simulink model "Controllo_Totale"  (R2013a)
settings: Solver=ode45  StartTime=0.0  StopTime=inf  RelTol=1e-3
undefined symbols (not defined in the file or in its folder): d, r
libraries: simulink x9, dspsigops x8, arduino_io_lib x6, xpcseriallib x2, dspnetwork x2
settings Model: Creator=Francesco  LastModifiedBy=Francesco

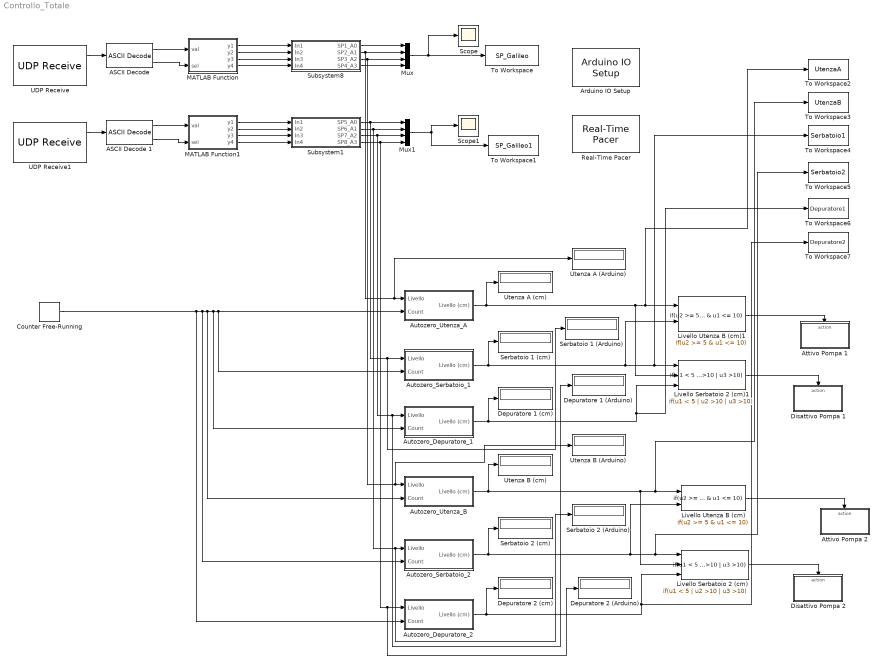
== system Controllo_Totale ==
  "ASCII Decode " : xpcseriallib/ASCII Decode   format=%d*%d\r  nvars=2  vartypes={ }
  ASCII Decode 1 : xpcseriallib/ASCII Decode   format=%d*%d\r  nvars=2  vartypes={ }
  Arduino IO Setup : arduino_io_lib/Arduino IO Setup  Priority=3  arduinoVar=Temporary arduino variable: Arduino1  workspaceVarName=a  comPort=COM3
  Attivo Pompa 1 : Subsystem  TreatAsAtomicUnit=on
  Attivo Pompa 2 : Subsystem  TreatAsAtomicUnit=on
  Autozero_Depuratore_1 : Subsystem
  Autozero_Depuratore_2 : Subsystem
  Autozero_Serbatoio_1 : Subsystem
  Autozero_Serbatoio_2 : Subsystem
  Autozero_Utenza_A : Subsystem
  Autozero_Utenza_B : Subsystem
  Counter Free-Running : simulink/Sources/Counter Free-Running  NumBits=32  tsamp=-1
  Depuratore 1 (Arduino) : Display
  Depuratore 1 (cm) : Display
  Depuratore 2 (Arduino) : Display
  Depuratore 2 (cm) : Display
  Disattivo Pompa 1 : Subsystem  TreatAsAtomicUnit=on
  Disattivo Pompa 2 : Subsystem  TreatAsAtomicUnit=on
  Livello Serbatoio 2 (cm) : If  NumInputs=3  IfExpression=u1 < 5 | u2 >10 | u3 >10  ShowElse=off
  Livello Serbatoio 2 (cm)1 : If  NumInputs=3  IfExpression=u1 < 5 | u2 >10 | u3 >10  ShowElse=off
  Livello Utenza B (cm) : If  NumInputs=2  IfExpression=u2 >= 5 & u1 <= 10  ShowElse=off
  Livello Utenza B (cm)1 : If  NumInputs=2  IfExpression=u2 >= 5 & u1 <= 10  ShowElse=off
  MATLAB Function : MATLAB Function  TreatAsAtomicUnit=on
  MATLAB Function1 : MATLAB Function  TreatAsAtomicUnit=on
  Mux : Mux
  Mux1 : Mux
  Real-Time Pacer : arduino_io_lib/Real-Time Pacer  simTimePerRealTime=1
  Scope : Scope
      settings: TimeRange=50  YMin=0  YMax=475
  Scope1 : Scope
      settings: TimeRange=50  YMin=327.5  YMax=360
  Serbatoio 1 (Arduino) : Display
  Serbatoio 1 (cm) : Display
  Serbatoio 2 (Arduino) : Display
  Serbatoio 2 (cm) : Display
  Subsystem1 : Subsystem
  Subsystem8 : Subsystem
  To Workspace : ToWorkspace  VariableName=SP_Galileo  SampleTime=-1  SaveFormat=Timeseries
  To Workspace1 : ToWorkspace  VariableName=SP_Galileo1  SampleTime=-1  SaveFormat=Timeseries
  To Workspace2 : ToWorkspace  VariableName=UtenzaA  SampleTime=-1
  To Workspace3 : ToWorkspace  VariableName=UtenzaB  SampleTime=-1
  To Workspace4 : ToWorkspace  VariableName=Serbatoio1  SampleTime=-1
  To Workspace5 : ToWorkspace  VariableName=Serbatoio2  SampleTime=-1
  To Workspace6 : ToWorkspace  VariableName=Depuratore1  SampleTime=-1
  To Workspace7 : ToWorkspace  VariableName=Depuratore2  SampleTime=-1
  UDP Receive : dspnetwork/UDP Receive  localURL='0.0.0.0'  localPort=4040  remoteURL='192.168.2.4'  remotePort=-1  recvBufferSize=1  dims=5  signalDatatype=uint8  isVarSize=off  showBlockingTime=on  blockingTime=inf  sampletime=1  blockPlatform=LINUX
  UDP Receive1 : dspnetwork/UDP Receive  localURL='0.0.0.0'  localPort=4040  remoteURL='192.168.2.6'  remotePort=-1  recvBufferSize=1  dims=5  signalDatatype=uint8  isVarSize=off  showBlockingTime=on  blockingTime=inf  sampletime=1  blockPlatform=LINUX
  Utenza A (Arduino) : Display
  Utenza A (cm) : Display
  Utenza B (Arduino) : Display
  Utenza B (cm) : Display
  wires:
  UDP Receive/1 -> "ASCII Decode "/1
  "ASCII Decode "/1 -> MATLAB Function/1(val)
  "ASCII Decode "/2 -> MATLAB Function/2(sel)
  Mux/1 -> To Workspace/1, Scope/1
  UDP Receive1/1 -> ASCII Decode 1/1
  ASCII Decode 1/1 -> MATLAB Function1/1(val)
  ASCII Decode 1/2 -> MATLAB Function1/2(sel)
  Mux1/1 -> To Workspace1/1, Scope1/1
  MATLAB Function/1(y1) -> Subsystem8/1(In1)
  MATLAB Function/2(y2) -> Subsystem8/2(In2)
  MATLAB Function/3(y3) -> Subsystem8/3(In3)
  MATLAB Function/4(y4) -> Subsystem8/4(In4)
  Subsystem8/1(SP1_A0) -> Mux/1
  Subsystem8/2(SP2_A1) -> Utenza A (Arduino)/1, Autozero_Utenza_A/1(Livello), Mux/2
  Subsystem8/3(SP3_A2) -> Utenza B (Arduino)/1, Autozero_Utenza_B/1(Livello), Mux/3
  Subsystem8/4(SP4_A3) -> Mux/4
  MATLAB Function1/1(y1) -> Subsystem1/1(In1)
  MATLAB Function1/2(y2) -> Subsystem1/2(In2)
  MATLAB Function1/3(y3) -> Subsystem1/3(In3)
  MATLAB Function1/4(y4) -> Subsystem1/4(In4)
  Subsystem1/1(SP5_A0) -> Autozero_Serbatoio_1/1(Livello), Serbatoio 1 (Arduino)/1, Mux1/1
  Subsystem1/2(SP6_A1) -> Serbatoio 2 (Arduino)/1, Autozero_Serbatoio_2/1(Livello), Mux1/2
  Subsystem1/3(SP7_A2) -> Depuratore 1 (Arduino)/1, Autozero_Depuratore_1/1(Livello), Mux1/3
  Subsystem1/4(SP8_A3) -> Depuratore 2 (Arduino)/1, Autozero_Depuratore_2/1(Livello), Mux1/4
  Autozero_Utenza_B/1(Livello (cm)) -> Livello Serbatoio 2 (cm)/2, To Workspace3/1, Livello Utenza B (cm)/1, Utenza B (cm)/1
  Counter Free-Running/1 -> Autozero_Depuratore_2/2(Count), Autozero_Utenza_A/2(Count), Autozero_Serbatoio_1/2(Count), Autozero_Depuratore_1/2(Count), Autozero_Utenza_B/2(Count), Autozero_Serbatoio_2/2(Count)
  Autozero_Serbatoio_2/1(Livello (cm)) -> Livello Utenza B (cm)/2, To Workspace5/1, Livello Serbatoio 2 (cm)/1, Serbatoio 2 (cm)/1
  Autozero_Depuratore_2/1(Livello (cm)) -> To Workspace7/1, Livello Serbatoio 2 (cm)/3, Depuratore 2 (cm)/1
  Livello Utenza B (cm)/1 -> Attivo Pompa 2/Action
  Livello Serbatoio 2 (cm)/1 -> Disattivo Pompa 2/Action
  Livello Utenza B (cm)1/1 -> Attivo Pompa 1/Action
  Livello Serbatoio 2 (cm)1/1 -> Disattivo Pompa 1/Action
  Autozero_Utenza_A/1(Livello (cm)) -> Utenza A (cm)/1, Livello Serbatoio 2 (cm)1/2, To Workspace2/1, Livello Utenza B (cm)1/1
  Autozero_Serbatoio_1/1(Livello (cm)) -> Serbatoio 1 (cm)/1, Livello Utenza B (cm)1/2, To Workspace4/1, Livello Serbatoio 2 (cm)1/1
  Autozero_Depuratore_1/1(Livello (cm)) -> Depuratore 1 (cm)/1, To Workspace6/1, Livello Serbatoio 2 (cm)1/3

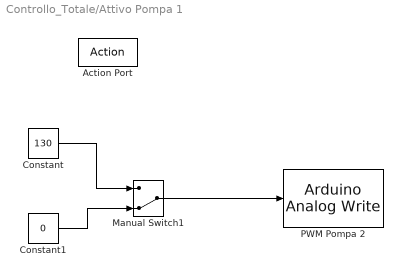
== system Controllo_Totale/Attivo Pompa 1 ==
  Action Port : ActionPort  ActionType=then
  Constant : Constant  Value=130
  Constant1 : Constant  Value=0  SampleTime=1
  Manual Switch1 : ManualSwitch  CurrentSetting=0
  PWM Pompa 2 : arduino_io_lib/Arduino Analog Write  arduinoVar=Temporary arduino variable: Arduino1  arduinoPin=5  T=1
  wires:
  Constant/1 -> Manual Switch1/1
  Constant1/1 -> Manual Switch1/2
  Manual Switch1/1 -> PWM Pompa 2/1

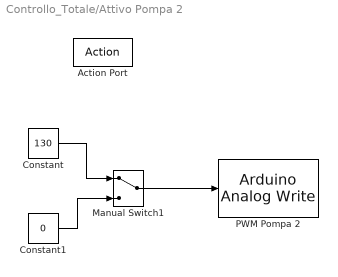
== system Controllo_Totale/Attivo Pompa 2 ==
  Action Port : ActionPort  ActionType=then
  Constant : Constant  Value=130
  Constant1 : Constant  Value=0  SampleTime=1
  Manual Switch1 : ManualSwitch
  PWM Pompa 2 : arduino_io_lib/Arduino Analog Write  arduinoVar=Temporary arduino variable: Arduino1  arduinoPin=6  T=1
  wires:
  Constant/1 -> Manual Switch1/1
  Constant1/1 -> Manual Switch1/2
  Manual Switch1/1 -> PWM Pompa 2/1

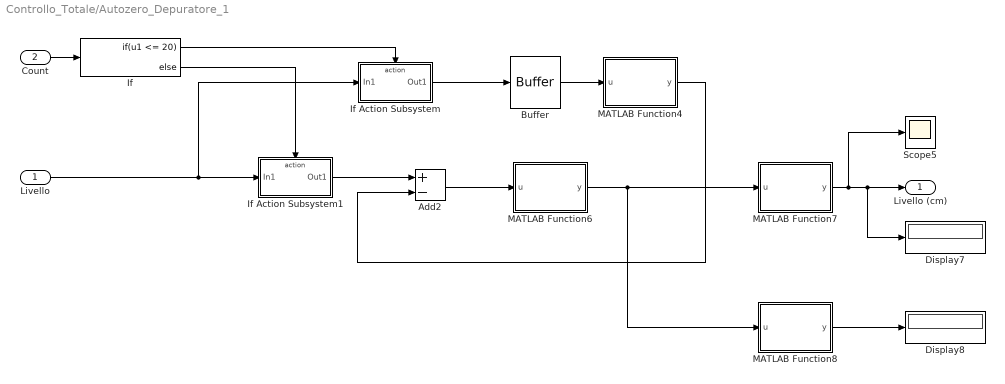
== system Controllo_Totale/Autozero_Depuratore_1 ==
  Livello : Inport
  Count : Inport  Port=2
  Add2 : Sum  Inputs=+-
  Buffer : Buffer  N=20  TreatMby1Signals=One channel
  Display7 : Display
  Display8 : Display
  If : If  IfExpression=u1 <= 20
  If Action Subsystem : Subsystem  TreatAsAtomicUnit=on
  If Action Subsystem1 : Subsystem  TreatAsAtomicUnit=on
  MATLAB Function4 : MATLAB Function  TreatAsAtomicUnit=on
  MATLAB Function6 : MATLAB Function  TreatAsAtomicUnit=on
  MATLAB Function7 : MATLAB Function  TreatAsAtomicUnit=on
  MATLAB Function8 : MATLAB Function  TreatAsAtomicUnit=on
  Scope5 : Scope
      settings: SaveName=ScopeData4
  Livello (cm) : Outport
  wires:
  Buffer/1 -> MATLAB Function4/1(u)
  MATLAB Function4/1(y) -> Add2/2
  If/1 -> If Action Subsystem/Action
  If/2 -> If Action Subsystem1/Action
  Add2/1 -> MATLAB Function6/1(u)
  MATLAB Function6/1(y) -> MATLAB Function8/1(u), MATLAB Function7/1(u)
  MATLAB Function8/1(y) -> Display8/1
  If Action Subsystem/1(Out1) -> Buffer/1
  MATLAB Function7/1(y) -> Display7/1, Livello (cm)/1, Scope5/1
  Count/1 -> If/1
  If Action Subsystem1/1(Out1) -> Add2/1
  Livello/1 -> If Action Subsystem/1(In1), If Action Subsystem1/1(In1)

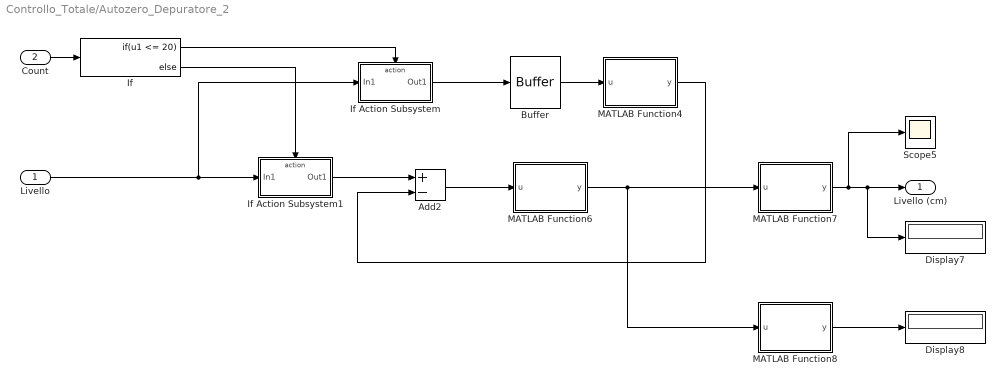
== system Controllo_Totale/Autozero_Depuratore_2 ==
  Livello : Inport
  Count : Inport  Port=2
  Add2 : Sum  Inputs=+-
  Buffer : Buffer  N=20  TreatMby1Signals=One channel
  Display7 : Display
  Display8 : Display
  If : If  IfExpression=u1 <= 20
  If Action Subsystem : Subsystem  TreatAsAtomicUnit=on
  If Action Subsystem1 : Subsystem  TreatAsAtomicUnit=on
  MATLAB Function4 : MATLAB Function  TreatAsAtomicUnit=on
  MATLAB Function6 : MATLAB Function  TreatAsAtomicUnit=on
  MATLAB Function7 : MATLAB Function  TreatAsAtomicUnit=on
  MATLAB Function8 : MATLAB Function  TreatAsAtomicUnit=on
  Scope5 : Scope
      settings: SaveName=ScopeData7
  Livello (cm) : Outport
  wires:
  Buffer/1 -> MATLAB Function4/1(u)
  MATLAB Function4/1(y) -> Add2/2
  If/1 -> If Action Subsystem/Action
  If/2 -> If Action Subsystem1/Action
  Add2/1 -> MATLAB Function6/1(u)
  MATLAB Function6/1(y) -> MATLAB Function8/1(u), MATLAB Function7/1(u)
  MATLAB Function8/1(y) -> Display8/1
  If Action Subsystem/1(Out1) -> Buffer/1
  MATLAB Function7/1(y) -> Display7/1, Livello (cm)/1, Scope5/1
  Count/1 -> If/1
  If Action Subsystem1/1(Out1) -> Add2/1
  Livello/1 -> If Action Subsystem/1(In1), If Action Subsystem1/1(In1)

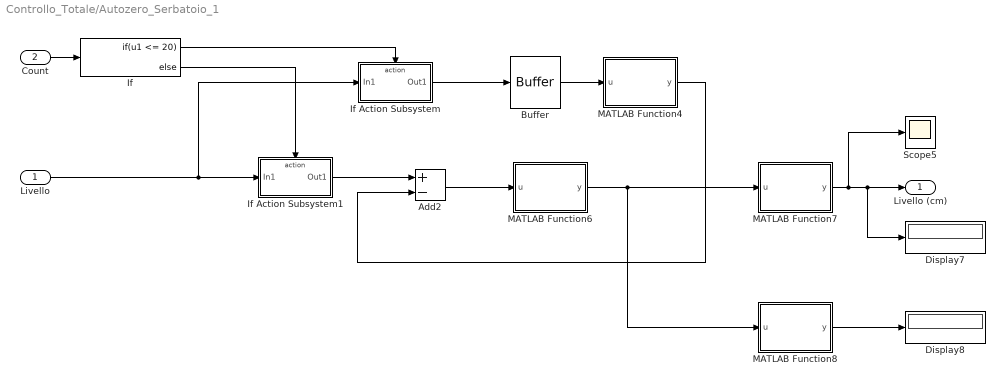
== system Controllo_Totale/Autozero_Serbatoio_1 ==
  Livello : Inport
  Count : Inport  Port=2
  Add2 : Sum  Inputs=+-
  Buffer : Buffer  N=20  TreatMby1Signals=One channel
  Display7 : Display
  Display8 : Display
  If : If  IfExpression=u1 <= 20
  If Action Subsystem : Subsystem  TreatAsAtomicUnit=on
  If Action Subsystem1 : Subsystem  TreatAsAtomicUnit=on
  MATLAB Function4 : MATLAB Function  TreatAsAtomicUnit=on
  MATLAB Function6 : MATLAB Function  TreatAsAtomicUnit=on
  MATLAB Function7 : MATLAB Function  TreatAsAtomicUnit=on
  MATLAB Function8 : MATLAB Function  TreatAsAtomicUnit=on
  Scope5 : Scope
      settings: SaveName=ScopeData2
  Livello (cm) : Outport
  wires:
  Buffer/1 -> MATLAB Function4/1(u)
  MATLAB Function4/1(y) -> Add2/2
  If/1 -> If Action Subsystem/Action
  If/2 -> If Action Subsystem1/Action
  Add2/1 -> MATLAB Function6/1(u)
  MATLAB Function6/1(y) -> MATLAB Function8/1(u), MATLAB Function7/1(u)
  MATLAB Function8/1(y) -> Display8/1
  If Action Subsystem/1(Out1) -> Buffer/1
  MATLAB Function7/1(y) -> Display7/1, Livello (cm)/1, Scope5/1
  Count/1 -> If/1
  If Action Subsystem1/1(Out1) -> Add2/1
  Livello/1 -> If Action Subsystem/1(In1), If Action Subsystem1/1(In1)

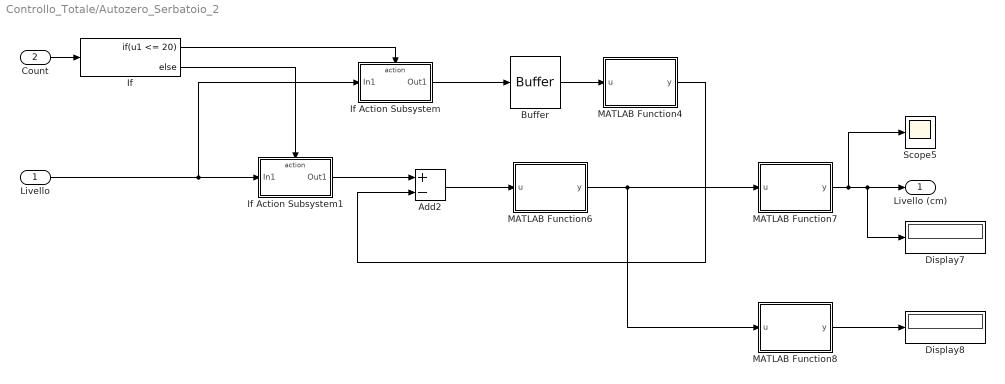
== system Controllo_Totale/Autozero_Serbatoio_2 ==
  Livello : Inport
  Count : Inport  Port=2
  Add2 : Sum  Inputs=+-
  Buffer : Buffer  N=20  TreatMby1Signals=One channel
  Display7 : Display
  Display8 : Display
  If : If  IfExpression=u1 <= 20
  If Action Subsystem : Subsystem  TreatAsAtomicUnit=on
  If Action Subsystem1 : Subsystem  TreatAsAtomicUnit=on
  MATLAB Function4 : MATLAB Function  TreatAsAtomicUnit=on
  MATLAB Function6 : MATLAB Function  TreatAsAtomicUnit=on
  MATLAB Function7 : MATLAB Function  TreatAsAtomicUnit=on
  MATLAB Function8 : MATLAB Function  TreatAsAtomicUnit=on
  Scope5 : Scope
      settings: SaveName=ScopeData6
  Livello (cm) : Outport
  wires:
  Buffer/1 -> MATLAB Function4/1(u)
  MATLAB Function4/1(y) -> Add2/2
  If/1 -> If Action Subsystem/Action
  If/2 -> If Action Subsystem1/Action
  Add2/1 -> MATLAB Function6/1(u)
  MATLAB Function6/1(y) -> MATLAB Function8/1(u), MATLAB Function7/1(u)
  MATLAB Function8/1(y) -> Display8/1
  If Action Subsystem/1(Out1) -> Buffer/1
  MATLAB Function7/1(y) -> Display7/1, Livello (cm)/1, Scope5/1
  Count/1 -> If/1
  If Action Subsystem1/1(Out1) -> Add2/1
  Livello/1 -> If Action Subsystem/1(In1), If Action Subsystem1/1(In1)

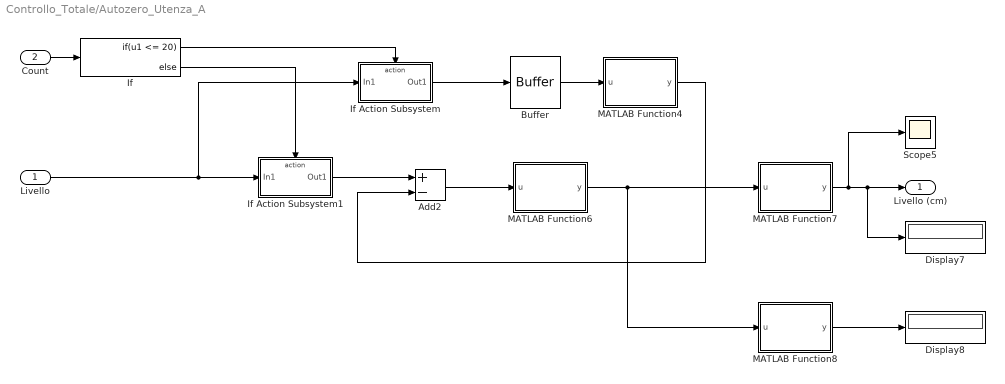
== system Controllo_Totale/Autozero_Utenza_A ==
  Livello : Inport
  Count : Inport  Port=2
  Add2 : Sum  Inputs=+-
  Buffer : Buffer  N=20  TreatMby1Signals=One channel
  Display7 : Display
  Display8 : Display
  If : If  IfExpression=u1 <= 20
  If Action Subsystem : Subsystem  TreatAsAtomicUnit=on
  If Action Subsystem1 : Subsystem  TreatAsAtomicUnit=on
  MATLAB Function4 : MATLAB Function  TreatAsAtomicUnit=on
  MATLAB Function6 : MATLAB Function  TreatAsAtomicUnit=on
  MATLAB Function7 : MATLAB Function  TreatAsAtomicUnit=on
  MATLAB Function8 : MATLAB Function  TreatAsAtomicUnit=on
  Scope5 : Scope
      settings: SaveName=ScopeData3
  Livello (cm) : Outport
  wires:
  Buffer/1 -> MATLAB Function4/1(u)
  MATLAB Function4/1(y) -> Add2/2
  If/1 -> If Action Subsystem/Action
  If/2 -> If Action Subsystem1/Action
  Add2/1 -> MATLAB Function6/1(u)
  MATLAB Function6/1(y) -> MATLAB Function8/1(u), MATLAB Function7/1(u)
  MATLAB Function8/1(y) -> Display8/1
  If Action Subsystem/1(Out1) -> Buffer/1
  MATLAB Function7/1(y) -> Display7/1, Livello (cm)/1, Scope5/1
  Count/1 -> If/1
  If Action Subsystem1/1(Out1) -> Add2/1
  Livello/1 -> If Action Subsystem/1(In1), If Action Subsystem1/1(In1)

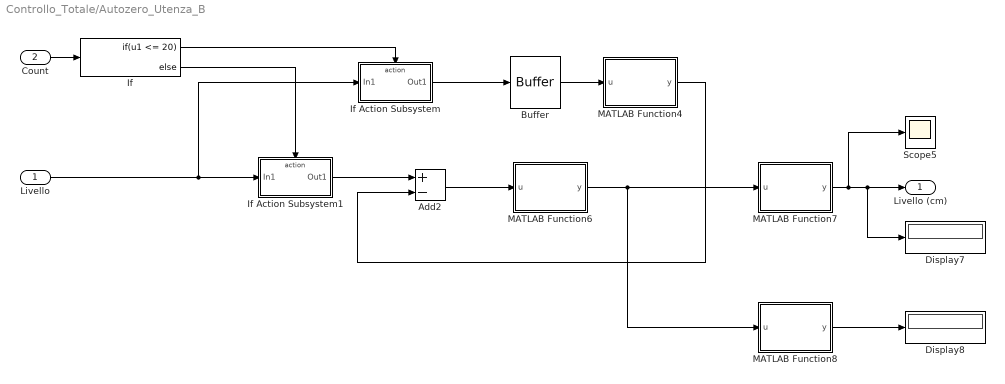
== system Controllo_Totale/Autozero_Utenza_B ==
  Livello : Inport
  Count : Inport  Port=2
  Add2 : Sum  Inputs=+-
  Buffer : Buffer  N=20  TreatMby1Signals=One channel
  Display7 : Display
  Display8 : Display
  If : If  IfExpression=u1 <= 20
  If Action Subsystem : Subsystem  TreatAsAtomicUnit=on
  If Action Subsystem1 : Subsystem  TreatAsAtomicUnit=on
  MATLAB Function4 : MATLAB Function  TreatAsAtomicUnit=on
  MATLAB Function6 : MATLAB Function  TreatAsAtomicUnit=on
  MATLAB Function7 : MATLAB Function  TreatAsAtomicUnit=on
  MATLAB Function8 : MATLAB Function  TreatAsAtomicUnit=on
  Scope5 : Scope
      settings: SaveName=ScopeData5
  Livello (cm) : Outport
  wires:
  Buffer/1 -> MATLAB Function4/1(u)
  MATLAB Function4/1(y) -> Add2/2
  If/1 -> If Action Subsystem/Action
  If/2 -> If Action Subsystem1/Action
  Add2/1 -> MATLAB Function6/1(u)
  MATLAB Function6/1(y) -> MATLAB Function8/1(u), MATLAB Function7/1(u)
  MATLAB Function8/1(y) -> Display8/1
  If Action Subsystem/1(Out1) -> Buffer/1
  MATLAB Function7/1(y) -> Display7/1, Livello (cm)/1, Scope5/1
  Count/1 -> If/1
  If Action Subsystem1/1(Out1) -> Add2/1
  Livello/1 -> If Action Subsystem/1(In1), If Action Subsystem1/1(In1)

== system Controllo_Totale/Disattivo Pompa 1 ==
  Action Port : ActionPort  ActionType=then
  Constant : Constant  Value=0
  PWM Pompa 1 : arduino_io_lib/Arduino Analog Write  arduinoVar=Temporary arduino variable: Arduino1  arduinoPin=5  T=1
  wires:
  Constant/1 -> PWM Pompa 1/1

== system Controllo_Totale/Disattivo Pompa 2 ==
  Action Port : ActionPort  ActionType=then
  Constant : Constant  Value=0
  PWM Pompa 2 : arduino_io_lib/Arduino Analog Write  arduinoVar=Temporary arduino variable: Arduino1  arduinoPin=6  T=1
  wires:
  Constant/1 -> PWM Pompa 2/1

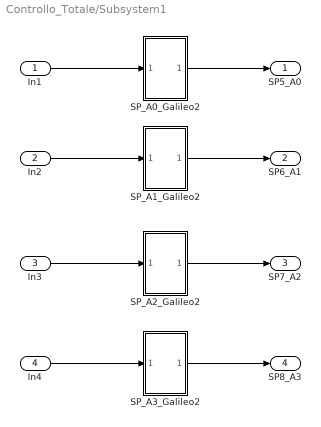
== system Controllo_Totale/Subsystem1 ==
  In1 : Inport
  In2 : Inport  Port=2
  In3 : Inport  Port=3
  In4 : Inport  Port=4
  SP_A0_Galileo2 : Subsystem
  SP_A1_Galileo2 : Subsystem
  SP_A2_Galileo2 : Subsystem
  SP_A3_Galileo2 : Subsystem
  SP5_A0 : Outport
  SP6_A1 : Outport  Port=2
  SP7_A2 : Outport  Port=3
  SP8_A3 : Outport  Port=4
  wires:
  In1/1 -> SP_A0_Galileo2/1(In1)
  In2/1 -> SP_A1_Galileo2/1(In1)
  In3/1 -> SP_A2_Galileo2/1(In1)
  In4/1 -> SP_A3_Galileo2/1(In1)
  SP_A0_Galileo2/1(Out1) -> SP5_A0/1
  SP_A1_Galileo2/1(Out1) -> SP6_A1/1
  SP_A2_Galileo2/1(Out1) -> SP7_A2/1
  SP_A3_Galileo2/1(Out1) -> SP8_A3/1

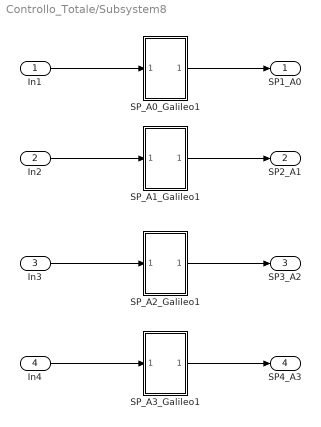
== system Controllo_Totale/Subsystem8 ==
  In1 : Inport
  In2 : Inport  Port=2
  In3 : Inport  Port=3
  In4 : Inport  Port=4
  SP_A0_Galileo1 : Subsystem
  SP_A1_Galileo1 : Subsystem
  SP_A2_Galileo1 : Subsystem
  SP_A3_Galileo1 : Subsystem
  SP1_A0 : Outport
  SP2_A1 : Outport  Port=2
  SP3_A2 : Outport  Port=3
  SP4_A3 : Outport  Port=4
  wires:
  In1/1 -> SP_A0_Galileo1/1(In1)
  In2/1 -> SP_A1_Galileo1/1(In1)
  In3/1 -> SP_A2_Galileo1/1(In1)
  In4/1 -> SP_A3_Galileo1/1(In1)
  SP_A0_Galileo1/1(Out1) -> SP1_A0/1
  SP_A1_Galileo1/1(Out1) -> SP2_A1/1
  SP_A2_Galileo1/1(Out1) -> SP3_A2/1
  SP_A3_Galileo1/1(Out1) -> SP4_A3/1

== system Controllo_Totale/Autozero_Depuratore_1/If Action Subsystem ==
  In1 : Inport
  Action Port : ActionPort  ActionType=then
  Out1 : Outport  InitialOutput=[0]
  wires:
  In1/1 -> Out1/1

== system Controllo_Totale/Autozero_Depuratore_1/If Action Subsystem1 ==
  In1 : Inport
  Action Port : ActionPort  ActionType=else
  Out1 : Outport  InitialOutput=[0]
  wires:
  In1/1 -> Out1/1

== system Controllo_Totale/Autozero_Depuratore_2/If Action Subsystem ==
  In1 : Inport
  Action Port : ActionPort  ActionType=then
  Out1 : Outport  InitialOutput=[0]
  wires:
  In1/1 -> Out1/1

== system Controllo_Totale/Autozero_Depuratore_2/If Action Subsystem1 ==
  In1 : Inport
  Action Port : ActionPort  ActionType=else
  Out1 : Outport  InitialOutput=[0]
  wires:
  In1/1 -> Out1/1

== system Controllo_Totale/Autozero_Serbatoio_1/If Action Subsystem ==
  In1 : Inport
  Action Port : ActionPort  ActionType=then
  Out1 : Outport  InitialOutput=[0]
  wires:
  In1/1 -> Out1/1

== system Controllo_Totale/Autozero_Serbatoio_1/If Action Subsystem1 ==
  In1 : Inport
  Action Port : ActionPort  ActionType=else
  Out1 : Outport  InitialOutput=[0]
  wires:
  In1/1 -> Out1/1

== system Controllo_Totale/Autozero_Serbatoio_2/If Action Subsystem ==
  In1 : Inport
  Action Port : ActionPort  ActionType=then
  Out1 : Outport  InitialOutput=[0]
  wires:
  In1/1 -> Out1/1

== system Controllo_Totale/Autozero_Serbatoio_2/If Action Subsystem1 ==
  In1 : Inport
  Action Port : ActionPort  ActionType=else
  Out1 : Outport  InitialOutput=[0]
  wires:
  In1/1 -> Out1/1

== system Controllo_Totale/Autozero_Utenza_A/If Action Subsystem ==
  In1 : Inport
  Action Port : ActionPort  ActionType=then
  Out1 : Outport  InitialOutput=[0]
  wires:
  In1/1 -> Out1/1

== system Controllo_Totale/Autozero_Utenza_A/If Action Subsystem1 ==
  In1 : Inport
  Action Port : ActionPort  ActionType=else
  Out1 : Outport  InitialOutput=[0]
  wires:
  In1/1 -> Out1/1

== system Controllo_Totale/Autozero_Utenza_B/If Action Subsystem ==
  In1 : Inport
  Action Port : ActionPort  ActionType=then
  Out1 : Outport  InitialOutput=[0]
  wires:
  In1/1 -> Out1/1

== system Controllo_Totale/Autozero_Utenza_B/If Action Subsystem1 ==
  In1 : Inport
  Action Port : ActionPort  ActionType=else
  Out1 : Outport  InitialOutput=[0]
  wires:
  In1/1 -> Out1/1

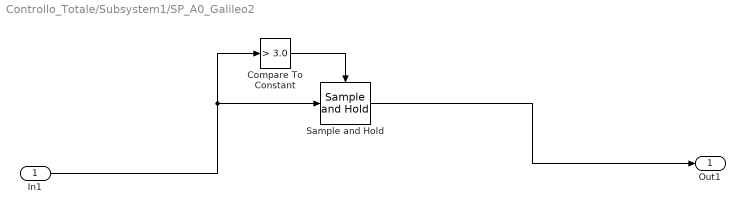
== system Controllo_Totale/Subsystem1/SP_A0_Galileo2 ==
  In1 : Inport
  Compare To Constant : simulink/Logic and Bit Operations/Compare To Constant  relop=>  const=3.0  OutDataTypeStr=boolean
  Sample and Hold : dspsigops/Sample and Hold  trig=Rising edge  initCond=0  latchinput=off
  Out1 : Outport
  wires:
  Sample and Hold/1 -> Out1/1
  In1/1 -> Compare To Constant/1, Sample and Hold/1
  Compare To Constant/1 -> Sample and Hold/Trigger

== system Controllo_Totale/Subsystem1/SP_A1_Galileo2 ==
  In1 : Inport
  Compare To Constant : simulink/Logic and Bit Operations/Compare To Constant  relop=>  const=3.0  OutDataTypeStr=boolean
  Sample and Hold : dspsigops/Sample and Hold  trig=Rising edge  initCond=0  latchinput=off
  Out1 : Outport
  wires:
  Sample and Hold/1 -> Out1/1
  In1/1 -> Compare To Constant/1, Sample and Hold/1
  Compare To Constant/1 -> Sample and Hold/Trigger

== system Controllo_Totale/Subsystem1/SP_A2_Galileo2 ==
  In1 : Inport
  Compare To Constant : simulink/Logic and Bit Operations/Compare To Constant  relop=>  const=3.0  OutDataTypeStr=boolean
  Sample and Hold : dspsigops/Sample and Hold  trig=Rising edge  initCond=0  latchinput=off
  Out1 : Outport
  wires:
  Sample and Hold/1 -> Out1/1
  In1/1 -> Compare To Constant/1, Sample and Hold/1
  Compare To Constant/1 -> Sample and Hold/Trigger

== system Controllo_Totale/Subsystem1/SP_A3_Galileo2 ==
  In1 : Inport
  Compare To Constant : simulink/Logic and Bit Operations/Compare To Constant  relop=>  const=3.0  OutDataTypeStr=boolean
  Sample and Hold : dspsigops/Sample and Hold  trig=Rising edge  initCond=0  latchinput=off
  Out1 : Outport
  wires:
  Sample and Hold/1 -> Out1/1
  In1/1 -> Compare To Constant/1, Sample and Hold/1
  Compare To Constant/1 -> Sample and Hold/Trigger

== system Controllo_Totale/Subsystem8/SP_A0_Galileo1 ==
  In1 : Inport
  Compare To Constant : simulink/Logic and Bit Operations/Compare To Constant  relop=>  const=3.0  OutDataTypeStr=boolean
  Sample and Hold : dspsigops/Sample and Hold  trig=Rising edge  initCond=0  latchinput=off
  Out1 : Outport
  wires:
  Sample and Hold/1 -> Out1/1
  In1/1 -> Compare To Constant/1, Sample and Hold/1
  Compare To Constant/1 -> Sample and Hold/Trigger

== system Controllo_Totale/Subsystem8/SP_A1_Galileo1 ==
  In1 : Inport
  Compare To Constant : simulink/Logic and Bit Operations/Compare To Constant  relop=>  const=3.0  OutDataTypeStr=boolean
  Sample and Hold : dspsigops/Sample and Hold  trig=Rising edge  initCond=0  latchinput=off
  Out1 : Outport
  wires:
  Sample and Hold/1 -> Out1/1
  In1/1 -> Compare To Constant/1, Sample and Hold/1
  Compare To Constant/1 -> Sample and Hold/Trigger

== system Controllo_Totale/Subsystem8/SP_A2_Galileo1 ==
  In1 : Inport
  Compare To Constant : simulink/Logic and Bit Operations/Compare To Constant  relop=>  const=3.0  OutDataTypeStr=boolean
  Sample and Hold : dspsigops/Sample and Hold  trig=Rising edge  initCond=0  latchinput=off
  Out1 : Outport
  wires:
  Sample and Hold/1 -> Out1/1
  In1/1 -> Compare To Constant/1, Sample and Hold/1
  Compare To Constant/1 -> Sample and Hold/Trigger

== system Controllo_Totale/Subsystem8/SP_A3_Galileo1 ==
  In1 : Inport
  Compare To Constant : simulink/Logic and Bit Operations/Compare To Constant  relop=>  const=3.0  OutDataTypeStr=boolean
  Sample and Hold : dspsigops/Sample and Hold  trig=Rising edge  initCond=0  latchinput=off
  Out1 : Outport
  wires:
  Sample and Hold/1 -> Out1/1
  In1/1 -> Compare To Constant/1, Sample and Hold/1
  Compare To Constant/1 -> Sample and Hold/Trigger

== matlab function Controllo_Totale/MATLAB Function1 ==
  data: val input; y1 output; sel input; y2 output; y3 output; y4 output
function [y1,y2,y3,y4] = fcn(val,sel)

y1=NaN;
y2=NaN;
y3=NaN;
y4=NaN;

if sel == 0
    y1 = val
end

if sel == 1
    y2 = val
end

if sel == 2
    y3 = val
end

if sel == 3
    y4 = val
end

== matlab function Controllo_Totale/MATLAB Function ==
  data: val input; y1 output; sel input; y2 output; y3 output; y4 output
function [y1,y2,y3,y4] = fcn(val,sel)

y1=NaN;
y2=NaN;
y3=NaN;
y4=NaN;

if sel == 0
    y1 = val
end

if sel == 1
    y2 = val
end

if sel == 2
    y3 = val
end

if sel == 3
    y4 = val
end

== matlab function Controllo_Totale/Autozero_Serbatoio_1/MATLAB Function4 ==
  data: u input; y output
function y = fcn(u)
%#codegen

%disp(u);

y = mode(u);

== matlab function Controllo_Totale/Autozero_Serbatoio_1/MATLAB Function6 ==
  data: u input; y output
function y = fcn(u)
%#codegen

if u < 0
    u = 0;
end

y = u;

== matlab function Controllo_Totale/Autozero_Utenza_A/MATLAB Function4 ==
  data: u input; y output
function y = fcn(u)
%#codegen

%disp(u);

y = mode(u);

== matlab function Controllo_Totale/Autozero_Serbatoio_1/MATLAB Function7 ==
  data: u input; y output
function y = volt2cm(u)
%#codegen

       p1 =  -2.863e-08;
       p2 =  -4.381e-06;
       p3 =      0.0426;
       p4 =  -4.632e-15;

y = p1 * u^3 + p2 * u^2 + p3 * u + p4;

if(y == p4)
    y = 0;
end

== matlab function Controllo_Totale/Autozero_Utenza_A/MATLAB Function6 ==
  data: u input; y output
function y = fcn(u)
%#codegen

if u < 0
    u = 0;
end

y = u;

== matlab function Controllo_Totale/Autozero_Utenza_A/MATLAB Function7 ==
  data: u input; y output
function y = volt2cm(u)
%#codegen

p1 =    1.16e-07;
p2 =  -9.339e-05;
p3 =     0.05238;
p4 =   2.776e-16;

y = p1 * u^3 + p2 * u^2 + p3 * u + p4;

if(y == p4)
    y = 0;
end

== matlab function Controllo_Totale/Autozero_Utenza_A/MATLAB Function8 ==
  data: u input; y output
function y = volt2ml(u)
%#codegen

p1 = 0.001123;

p2 = -0.2136;

p3 = 26.88;

p4 = 0;


y = p1 * u^3 + p2 * u^2 + p3 * u + p4;

== matlab function Controllo_Totale/Autozero_Serbatoio_1/MATLAB Function8 ==
  data: u input; y output
function y = volt2ml(u)
%#codegen

p1 = 0.001123;

p2 = -0.2136;

p3 = 26.88;

p4 = 0;


y = p1 * u^3 + p2 * u^2 + p3 * u + p4;

== matlab function Controllo_Totale/Autozero_Depuratore_1/MATLAB Function4 ==
  data: u input; y output
function y = fcn(u)
%#codegen

%disp(u);

y = mode(u);

== matlab function Controllo_Totale/Autozero_Depuratore_1/MATLAB Function6 ==
  data: u input; y output
function y = fcn(u)
%#codegen

if u < 0
    u = 0;
end

y = u;

== matlab function Controllo_Totale/Autozero_Depuratore_1/MATLAB Function7 ==
  data: u input; y output
function y = volt2cm(u)
%#codegen

       p1 =   8.338e-08;
       p2 =  -7.011e-05;
       p3 =     0.05011;
       p4 =   5.048e-15;

y = p1 * u^3 + p2 * u^2 + p3 * u + p4;

if(y == p4)
    y = 0;
end

== matlab function Controllo_Totale/Autozero_Depuratore_1/MATLAB Function8 ==
  data: u input; y output
function y = volt2ml(u)
%#codegen

p1 = 0.001123;

p2 = -0.2136;

p3 = 26.88;

p4 = 0;


y = p1 * u^3 + p2 * u^2 + p3 * u + p4;

== matlab function Controllo_Totale/Autozero_Utenza_B/MATLAB Function4 ==
  data: u input; y output
function y = fcn(u)
%#codegen

%disp(u);

y = mode(u);

== matlab function Controllo_Totale/Autozero_Utenza_B/MATLAB Function6 ==
  data: u input; y output
function y = fcn(u)
%#codegen

if u < 0
    u = 0;
end

y = u;

== matlab function Controllo_Totale/Autozero_Utenza_B/MATLAB Function7 ==
  data: u input; y output
function y = volt2cm(u)
%#codegen

p1 =   2.013e-07;
p2 =  -0.0001372;
p3 =     0.05877;
p4 =   3.903e-15;

y = p1 * u^3 + p2 * u^2 + p3 * u + p4;

if(y == p4)
    y = 0;
end

== matlab function Controllo_Totale/Autozero_Utenza_B/MATLAB Function8 ==
  data: u input; y output
function y = volt2ml(u)
%#codegen

p1 = 0.001123;

p2 = -0.2136;

p3 = 26.88;

p4 = 0;


y = p1 * u^3 + p2 * u^2 + p3 * u + p4;

== matlab function Controllo_Totale/Autozero_Serbatoio_2/MATLAB Function4 ==
  data: u input; y output
function y = fcn(u)
%#codegen

%disp(u);

y = mode(u);

== matlab function Controllo_Totale/Autozero_Serbatoio_2/MATLAB Function6 ==
  data: u input; y output
function y = fcn(u)
%#codegen

if u < 0
    u = 0;
end

y = u;

== matlab function Controllo_Totale/Autozero_Serbatoio_2/MATLAB Function7 ==
  data: u input; y output
function y = volt2cm(u)
%#codegen

       p1 =   4.143e-08;
       p2 =  -4.221e-05;
       p3 =     0.04614;
       p4 =   1.735e-17;

y = p1 * u^3 + p2 * u^2 + p3 * u + p4;

if(y == p4)
    y = 0;
end

== matlab function Controllo_Totale/Autozero_Serbatoio_2/MATLAB Function8 ==
  data: u input; y output
function y = volt2ml(u)
%#codegen

p1 = 0.001123;

p2 = -0.2136;

p3 = 26.88;

p4 = 0;


y = p1 * u^3 + p2 * u^2 + p3 * u + p4;

== matlab function Controllo_Totale/Autozero_Depuratore_2/MATLAB Function4 ==
  data: u input; y output
function y = fcn(u)
%#codegen

%disp(u);

y = mode(u);

== matlab function Controllo_Totale/Autozero_Depuratore_2/MATLAB Function6 ==
  data: u input; y output
function y = fcn(u)
%#codegen

if u < 0
    u = 0;
end

y = u;

== matlab function Controllo_Totale/Autozero_Depuratore_2/MATLAB Function7 ==
  data: u input; y output
function y = volt2cm(u)
%#codegen

       p1 =   7.848e-08;
       p2 =  -5.702e-05;
       p3 =     0.04508;
       p4 =  -3.938e-15;

y = p1 * u^3 + p2 * u^2 + p3 * u + p4;

if(y == p4)
    y = 0;
end

== matlab function Controllo_Totale/Autozero_Depuratore_2/MATLAB Function8 ==
  data: u input; y output
function y = volt2ml(u)
%#codegen

p1 = 0.001123;

p2 = -0.2136;

p3 = 26.88;

p4 = 0;


y = p1 * u^3 + p2 * u^2 + p3 * u + p4;
